simulink model "Simulink_Simulink_PIL_Cruise_Crontrol_r2020b"  (R2024a)
settings: Solver=VariableStepAuto  StartTime=0.0  StopTime=Tsim  FixedStep=Ts/20  RelTol=1e-3
values from neighbouring files (symbols this model uses):
  noise = 0    [main_Simulink_PIL_Cruise_Crontrol.m]
  PIL = 1    [main_Simulink_PIL_Cruise_Crontrol.m]
  Ts = 1/fs    (= 0.01)    [main_Simulink_PIL_Cruise_Crontrol.m]
undefined symbols (not defined in the file or in its folder): g
libraries: aerolibactuator x2, aerolibatmos2 x2, simulink x1
settings Model: SimulationMode=accelerator  Creator=ricardo  LastModifiedBy=mason
settings SolverCC: AlgebraicLoopSolver=TrustRegion
settings DataIOCC: ReturnWorkspaceOutputs=off
settings DebuggingCC: UnconnectedInputMsg=warning  UnconnectedOutputMsg=warning  UnconnectedLineMsg=warning  ArithmeticOperatorsInVariantConditions=warning
settings ModelReferenceCC: EnableRefExpFcnMdlSchedulingChecks=on
settings SFSimCC: CustomCodeUndefinedFunction=UseInterfaceOnly
settings RTWCC: GPUComputeCapability=3.5  DLArmComputeVersion=19.05

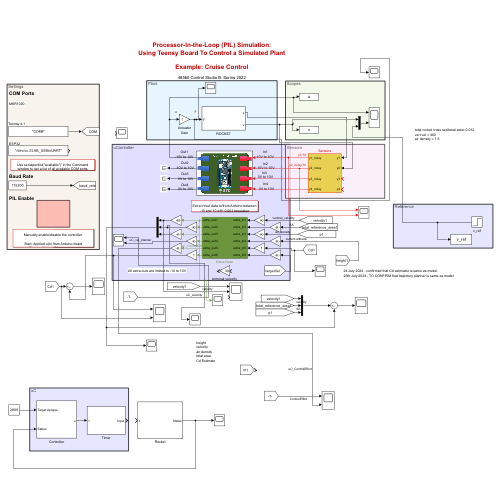
[thumbnail: Simulink's stored preview of the top-level diagram]
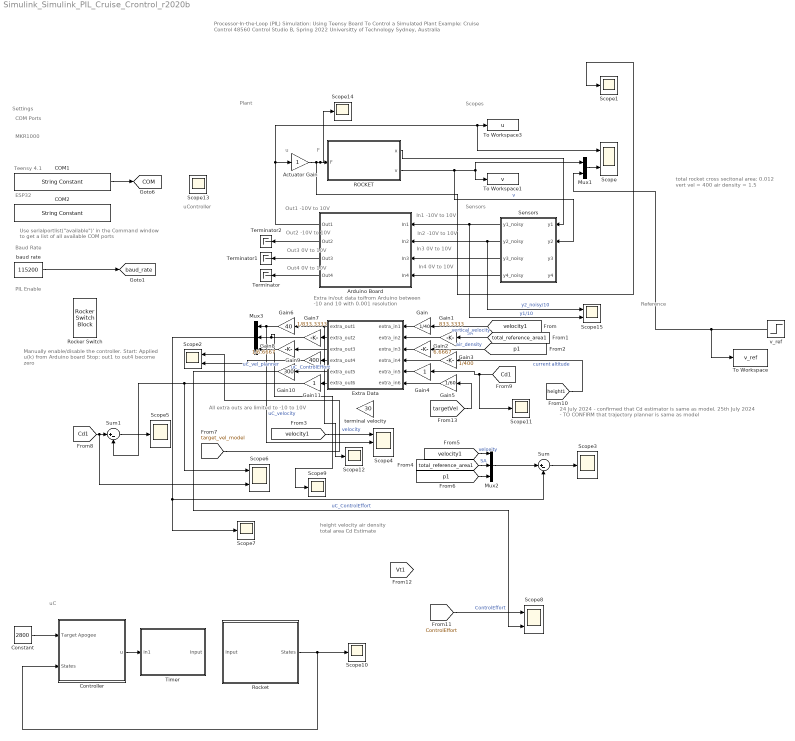
== system Simulink_Simulink_PIL_Cruise_Crontrol_r2020b ==
  note: 24 July 2024 - confirmed that Cd estimator is same as model.
      | 25th July 2024 - TO CONFIRM that trajectory planner is same as model
  note: All extra outs are limited to -10 to 10V
  note: height
      | velocity
      | air density
      | total area
      | Cd Estimate
  note: total rocket cross secitonal area: 0.012
      | vert vel = 400
      | air density = 1.5
  note: F
  note: u
  note: MKR1000
  note: COM Ports
  note: Settings
  note: Scopes
  note: Plant
  note: Reference
  note: Sensors
  note: uController
  note: Out1
      | -10V to 10V
  note: Processor-In-the-Loop (PIL) Simulation:
      | Using Teensy Board To Control a Simulated Plant
      |
      | Example: Cruise Control
      |
      | 48560 Control Studio B, Spring 2022
      | Universitty of Technology Sydney, Australia
  note: Out2
      | -10V to 10V
  note: Out3
      | 0V to 10V
  note: Out4
      | 0V to 10V
  note: In1
      | -10V to 10V
  note: In2
      | -10V to 10V
  note: In3
      | 0V to 10V
  note: In4
      | 0V to 10V
  note: Manually enable/disable the controller.
      |
      | Start: Applied u(k) from Arduino board
      | Stop: out1 to out4 become zero
  note: Extra in/out data to/from Arduino between -10 and 10 with 0.001 resolution
  note: Baud Rate
  note: PIL Enable
  note: Use serialportlist("available")' in the Command window to get a list of all available COM ports
  note: ESP32
  note: Teensy 4.1
  note: uC
  Actuator Gain : Gain
  Arduino Board : Subsystem
      mask Display: image('$imagefile'); % Use "Edit Image" on toolstrip to change.
  COM1 : StringConstant  String="\"COM8\""
  COM2 : StringConstant  String="\"/dev/cu.SLAB_USBtoUART\""
  Constant : Constant  Value=2800
  Controller : Subsystem
  Extra Data : Subsystem
  Gain : Gain  Gain=1/40
  Gain1 : Gain  Gain=833.3333
  Gain10 : Gain  Gain=300
  Gain11 : Gain
  Gain2 : Gain  Gain=6.6667
  Gain3 : Gain  Gain=1/400
  Gain4 : Gain
  Gain5 : Gain  Gain=1/60
  Gain6 : Gain  Gain=40
  Gain7 : Gain  Gain=1/833.3333
  Gain8 : Gain  Gain=1/6.6667
  Gain9 : Gain  Gain=400
  Mux1 : Mux  Inputs=2
  Mux2 : Mux  Inputs=3
  Mux3 : Mux  Inputs=3
  ROCKET : Subsystem
  Rocker Switch : RockerSwitchBlock  LabelPosition=Hide
      settings: Values={{'Stop', 'Start'}, [0 1]}
  Rocket : Subsystem
  Scope{,2,6,8,15} (5 alike) : Scope  NumInputPorts=2
  Scope{1,3,5,7,9..14} (10 alike) : Scope
  Scope4 : Scope  NumInputPorts=3
  Sensors : Subsystem
  Sum : Sum  Inputs=|+-
  Sum1 : Sum  Inputs=|+-
  Terminator : Terminator
  Terminator1 : Terminator
  Terminator2 : Terminator
  Timer : Subsystem
  To Workspace : ToWorkspace  VariableName=v_ref  SampleTime=Ts/20
  To Workspace1 : ToWorkspace  VariableName=v  SampleTime=Ts/20
  To Workspace3 : ToWorkspace  VariableName=u  SampleTime=Ts/20
  baud rate : Constant  Value=115200
  terminal velocity : Gain  Gain=30
  v_ref : Step  Time=0.001  After=2800  SampleTime=0
  tag scope: COM=global, baud_rate=global
  wires:
  Arduino Board/2(Out2) -> Terminator2/1
  Arduino Board/3(Out3) -> Terminator1/1
  Arduino Board/4(Out4) -> Terminator/1
  Extra Data/1(extra_out1) -> Gain6/1, Scope12/1
  Extra Data/3(extra_out3) -> Gain8/1
  Sensors/1(y1_noisy) -> Scope15/2, Arduino Board/1(In1)  "y1/10"
  Sensors/4(y4_noisy) -> Arduino Board/4(In4)
  baud rate/1 -> [baud_rate]
  Sensors/2(y2_noisy) -> Scope15/1, Arduino Board/2(In2)  "y2_noisy/10"
  Sensors/3(y3_noisy) -> Arduino Board/3(In3)
  v_ref/1 -> To Workspace/1, Mux1/2
  ROCKET/2(v) -> Mux1/1, To Workspace1/1, Sensors/2(y2)  "v"
  ROCKET/1(x) -> Sensors/1(y1)
  Actuator Gain/1 -> Scope14/1, ROCKET/1(F), Scope1/1
  Mux1/1 -> Scope/2
  COM1/1 -> [COM]
  Rocket/1(States) -> Scope10/1, Controller/2(States)
  Constant/1 -> Controller/1(Target Apogee)
  Controller/1(u) -> Timer/1(In1)
  Gain/1 -> Extra Data/1(extra_in1)
  Gain1/1 -> Extra Data/2(extra_in2)
  Gain2/1 -> Extra Data/3(extra_in3)
  Gain4/1 -> Extra Data/5(extra_in5)
  Gain3/1 -> Extra Data/4(extra_in4)
  Gain5/1 -> Extra Data/6(extra_in6)
  Gain9/1 -> Scope2/2  "uC_vel_planner"
  Gain8/1 -> Mux3/3
  Gain6/1 -> Scope4/2, Mux3/1  "uC_velocity"
  Extra Data/2(extra_out2) -> Gain7/1
  Extra Data/4(extra_out4) -> Gain9/1
  Extra Data/6(extra_out6) -> Gain11/1
  [total_reference_area1] -> Gain1/1  "SA"
  [velocity1] -> Gain/1  "vertical_velocity"
  [p1] -> Gain2/1  "air_density"
  [velocity1] -> Mux2/1  "velocity"
  [total_reference_area1] -> Mux2/2  "SA"
  [p1] -> Mux2/3
  Mux2/1 -> Sum/1
  Mux3/1 -> Scope7/1, Sum/2
  Sum/1 -> Scope3/1
  [velocity1] -> Scope4/1  "velocity"
  [Cd1] -> Scope6/2, Sum1/1
  Gain11/1 -> Scope6/1, Sum1/2
  Sum1/1 -> Scope5/1
  [height1] -> Gain3/1  "current altitude"
  [target_vel_model] -> Scope2/1
  Extra Data/5(extra_out5) -> Gain10/1  "uC_ControlEffort"
  Gain7/1 -> Scope9/1, Mux3/2
  [Cd1] -> Scope11/1, Gain4/1
  Arduino Board/1(Out1) -> Scope/1, To Workspace3/1, Actuator Gain/1
  [ControlEffort] -> Scope8/1  "ControlEffort"
  Gain10/1 -> Scope8/2  "uC_ControlEffort"
  [targetVel] -> Gain5/1

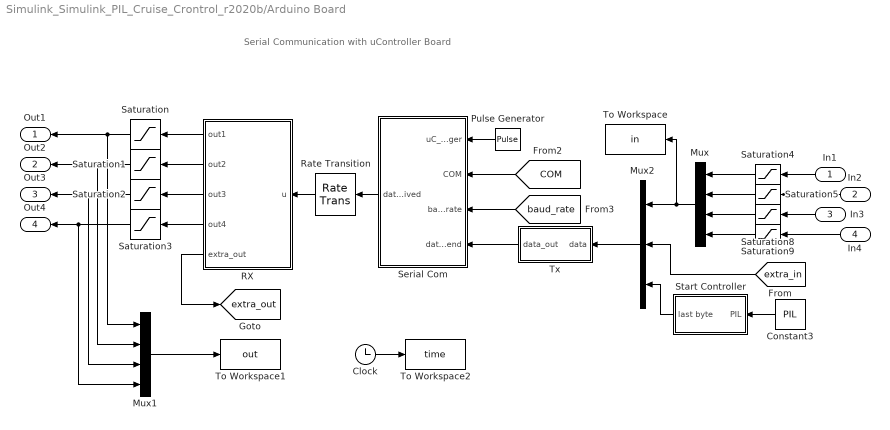
== system Simulink_Simulink_PIL_Cruise_Crontrol_r2020b/Arduino Board ==
  note: Serial Communication with uController Board
  In1 : Inport
  In2 : Inport  Port=2
  In3 : Inport  Port=3
  In4 : Inport  Port=4
  Clock : Clock
  Constant3 : Constant  Value=PIL
  Mux : Mux
  Mux1 : Mux
  Mux2 : Mux  Inputs=3
  Pulse Generator : DiscretePulseGenerator  PulseType=Time based  Period=Ts  PulseWidth=50
  RX : MATLAB Function  TreatAsAtomicUnit=on
  Rate Transition : RateTransition  InitialCondition=zeros(21,1)
  Saturation{,1,4..5} (4 alike) : Saturate  UpperLimit=10  LowerLimit=-10
  Saturation{2..3,8..9} (4 alike) : Saturate  UpperLimit=10  LowerLimit=0
  Serial Com : MATLAB Function  TreatAsAtomicUnit=on  SystemSampleTime=Ts/10
  Start Controller : Subsystem
  To Workspace : ToWorkspace  VariableName=in  SampleTime=Ts/20
  To Workspace1 : ToWorkspace  VariableName=out  SampleTime=Ts/20
  To Workspace2 : ToWorkspace  VariableName=time  SampleTime=Ts/20
  Tx : MATLAB Function  TreatAsAtomicUnit=on  SystemSampleTime=Ts/10
  Out1 : Outport  VectorParamsAs1DForOutWhenUnconnected=off
  Out2 : Outport  Port=2  VectorParamsAs1DForOutWhenUnconnected=off
  Out3 : Outport  Port=3  VectorParamsAs1DForOutWhenUnconnected=off
  Out4 : Outport  Port=4  VectorParamsAs1DForOutWhenUnconnected=off
  tag scope: extra_out=global
  wires:
  RX/1(out1) -> Saturation/1
  RX/2(out2) -> Saturation1/1
  RX/3(out3) -> Saturation2/1
  Mux1/1 -> To Workspace1/1
  Clock/1 -> To Workspace2/1
  Saturation/1 -> Out1/1, Mux1/1
  Saturation1/1 -> Out2/1, Mux1/2
  Saturation2/1 -> Out3/1, Mux1/3
  Saturation3/1 -> Out4/1, Mux1/4
  RX/4(out4) -> Saturation3/1
  RX/5(extra_out) -> [extra_out]
  Mux/1 -> Mux2/1, To Workspace/1
  [COM] -> Serial Com/2(COM)
  [baud_rate] -> Serial Com/3(baud_rate)
  Pulse Generator/1 -> Serial Com/1(uC_trigger)
  Serial Com/1(data_received) -> Rate Transition/1
  Rate Transition/1 -> RX/1(u)
  Constant3/1 -> Start Controller/1(PIL)
  In1/1 -> Saturation4/1
  In2/1 -> Saturation5/1
  In3/1 -> Saturation8/1
  In4/1 -> Saturation9/1
  Saturation4/1 -> Mux/1
  Saturation5/1 -> Mux/2
  Saturation8/1 -> Mux/3
  Saturation9/1 -> Mux/4
  [extra_in] -> Mux2/2
  Start Controller/1(last byte) -> Mux2/3
  Mux2/1 -> Tx/1(data)
  Tx/1(data_out) -> Serial Com/4(data_send)

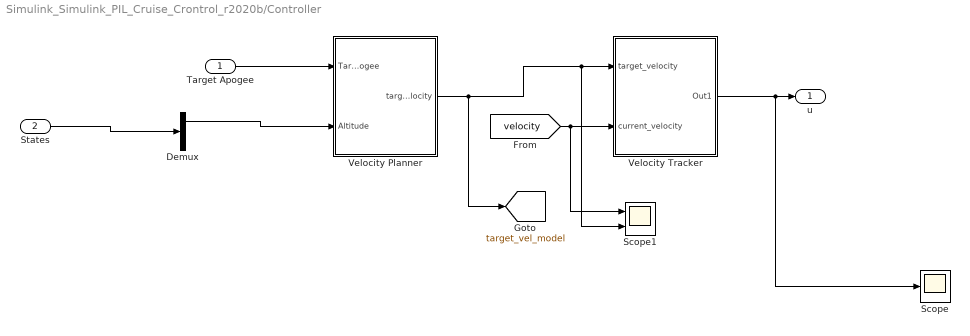
== system Simulink_Simulink_PIL_Cruise_Crontrol_r2020b/Controller ==
  Target Apogee : Inport
  States : Inport  Port=2
  Demux : Demux  Outputs=5
  Scope : Scope
  Scope1 : Scope  NumInputPorts=2
  Velocity Planner : Subsystem
  Velocity Tracker : Subsystem
  u : Outport
  tag scope: target_vel_model=global
  wires:
  Target Apogee/1 -> Velocity Planner/1(Target Apogee)
  Velocity Tracker/1(Out1) -> Scope/1, u/1
  [velocity] -> Scope1/1, Velocity Tracker/2(current_velocity)
  Velocity Planner/1(target_velocity) -> [target_vel_model], Scope1/2, Velocity Tracker/1(target_velocity)
  States/1 -> Demux/1
  Demux/1 -> Velocity Planner/2(Altitude)

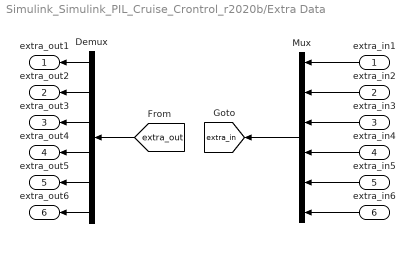
== system Simulink_Simulink_PIL_Cruise_Crontrol_r2020b/Extra Data ==
  extra_in1 : Inport
  extra_in2 : Inport  Port=2
  extra_in3 : Inport  Port=3
  extra_in4 : Inport  Port=4
  extra_in5 : Inport  Port=5
  extra_in6 : Inport  Port=6
  Demux : Demux  Outputs=6
  Mux : Mux  Inputs=6
  extra_out1 : Outport
  extra_out2 : Outport  Port=2
  extra_out3 : Outport  Port=3
  extra_out4 : Outport  Port=4
  extra_out5 : Outport  Port=5
  extra_out6 : Outport  Port=6
  tag scope: extra_in=global
  wires:
  extra_in4/1 -> Mux/4
  extra_in3/1 -> Mux/3
  extra_in2/1 -> Mux/2
  extra_in1/1 -> Mux/1
  Mux/1 -> [extra_in]
  [extra_out] -> Demux/1
  Demux/1 -> extra_out1/1
  Demux/2 -> extra_out2/1
  Demux/3 -> extra_out3/1
  Demux/4 -> extra_out4/1
  extra_in5/1 -> Mux/5
  extra_in6/1 -> Mux/6
  Demux/6 -> extra_out6/1
  Demux/5 -> extra_out5/1

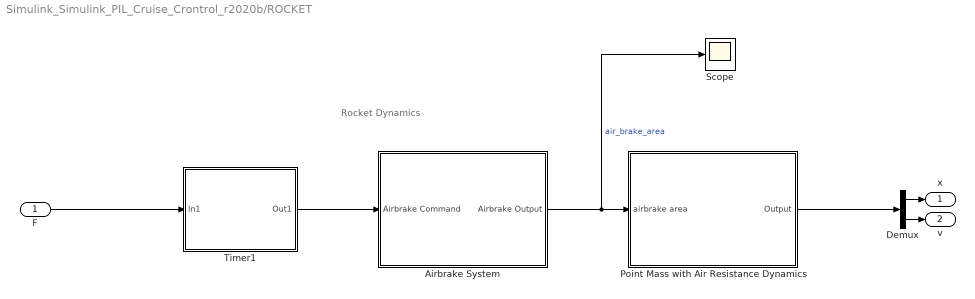
== system Simulink_Simulink_PIL_Cruise_Crontrol_r2020b/ROCKET ==
  note: Rocket Dynamics
  F : Inport
  Airbrake System : Subsystem
      mask Display: image('airbrake.png');
  Demux : Demux  Outputs=2
  "Point Mass with Air Resistance Dynamics " : Subsystem
      mask Display: image('rocket.jpeg');
  Scope : Scope
  Timer1 : Subsystem
  x : Outport  VectorParamsAs1DForOutWhenUnconnected=off
  v : Outport  Port=2  VectorParamsAs1DForOutWhenUnconnected=off
  wires:
  Airbrake System/1(Airbrake Output) -> Scope/1, "Point Mass with Air Resistance Dynamics "/1(airbrake area)  "air_brake_area"
  F/1 -> Timer1/1(In1)
  "Point Mass with Air Resistance Dynamics "/1(Output) -> Demux/1
  Demux/1 -> x/1
  Demux/2 -> v/1
  Timer1/1(Out1) -> Airbrake System/1(Airbrake Command)

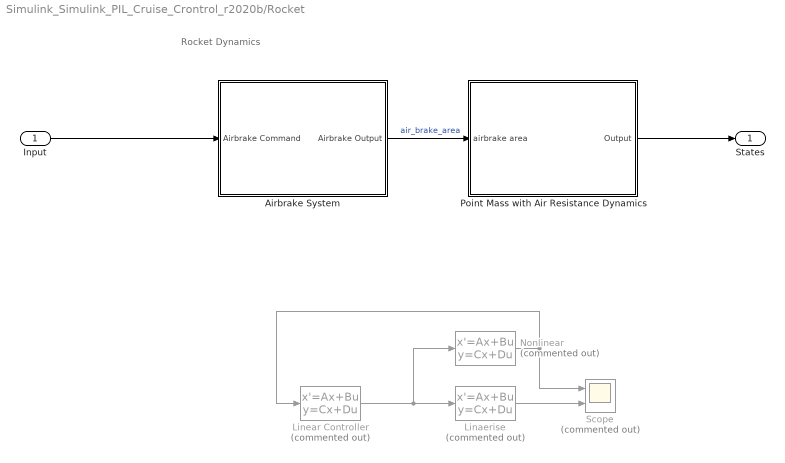
== system Simulink_Simulink_PIL_Cruise_Crontrol_r2020b/Rocket ==
  note: Rocket Dynamics
  Input : Inport
  Airbrake System : Subsystem
      mask Display: image('airbrake.png');
  "Linaerise " : StateSpace  Commented=on  InitialCondition=0
  Linear Controller : StateSpace  Commented=on  InitialCondition=0
  Nonlinear : StateSpace  Commented=on  InitialCondition=0
  "Point Mass with Air Resistance Dynamics " : Subsystem
      mask Display: image('rocket.jpeg');
  Scope : Scope  Commented=on  NumInputPorts=2
  States : Outport
  wires:
  "Point Mass with Air Resistance Dynamics "/1(Output) -> States/1
  Linear Controller/1 -> Nonlinear/1, "Linaerise "/1
  Nonlinear/1 -> Linear Controller/1, Scope/1
  "Linaerise "/1 -> Scope/2
  Input/1 -> Airbrake System/1(Airbrake Command)
  Airbrake System/1(Airbrake Output) -> "Point Mass with Air Resistance Dynamics "/1(airbrake area)  "air_brake_area"

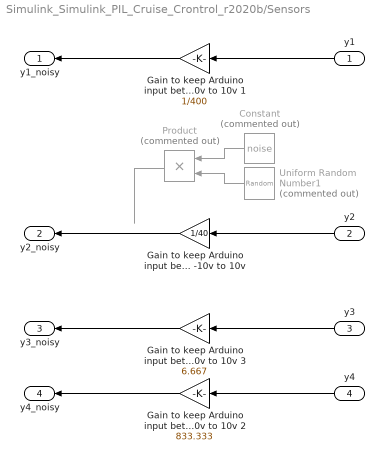
== system Simulink_Simulink_PIL_Cruise_Crontrol_r2020b/Sensors ==
  y1 : Inport
  y2 : Inport  Port=2
  y3 : Inport  Port=3
  y4 : Inport  Port=4
  Constant : Constant  Commented=on  Value=noise
  "Gain to keep Arduino input between -10v to 10v " : Gain  Gain=1/40
  Gain to keep Arduino input between -10v to 10v 1 : Gain  Gain=1/400
  Gain to keep Arduino input between -10v to 10v 2 : Gain  Gain=833.333
  Gain to keep Arduino input between -10v to 10v 3 : Gain  Gain=6.667
  Product : Product  Commented=on
  Uniform Random Number1 : UniformRandomNumber  Commented=on  Minimum=-0.1  Maximum=0.1  SampleTime=0.5*Ts
  y1_noisy : Outport  VectorParamsAs1DForOutWhenUnconnected=off
  y2_noisy : Outport  Port=2  VectorParamsAs1DForOutWhenUnconnected=off
  y3_noisy : Outport  Port=3  VectorParamsAs1DForOutWhenUnconnected=off
  y4_noisy : Outport  Port=4  VectorParamsAs1DForOutWhenUnconnected=off
  wires:
  y2/1 -> "Gain to keep Arduino input between -10v to 10v "/1
  y3/1 -> Gain to keep Arduino input between -10v to 10v 3/1
  y4/1 -> Gain to keep Arduino input between -10v to 10v 2/1
  y1/1 -> Gain to keep Arduino input between -10v to 10v 1/1
  Uniform Random Number1/1 -> Product/2
  Product/1 -> ?
  Constant/1 -> Product/1
  "Gain to keep Arduino input between -10v to 10v "/1 -> y2_noisy/1
  Gain to keep Arduino input between -10v to 10v 1/1 -> y1_noisy/1
  Gain to keep Arduino input between -10v to 10v 2/1 -> y4_noisy/1
  Gain to keep Arduino input between -10v to 10v 3/1 -> y3_noisy/1

== system Simulink_Simulink_PIL_Cruise_Crontrol_r2020b/Timer ==
  In1 : Inport
  Clock : Clock
  Constant1 : Constant  Value=0
  Switch : Switch  Criteria=u2 > Threshold  Threshold=5  SaturateOnIntegerOverflow=off  InputSameDT=off
  Input : Outport
  wires:
  Switch/1 -> Input/1
  Clock/1 -> Switch/2
  In1/1 -> Switch/1
  Constant1/1 -> Switch/3

== system Simulink_Simulink_PIL_Cruise_Crontrol_r2020b/Arduino Board/Start Controller ==
  PIL : Inport
  Constant : Constant  Value=0
  Constant1 : Constant  Value=255
  Switch : Switch  Criteria=u2 > Threshold  SaturateOnIntegerOverflow=off  InputSameDT=off
  last byte : Outport
  wires:
  Switch/1 -> last byte/1
  PIL/1 -> Switch/2
  Constant1/1 -> Switch/1
  Constant/1 -> Switch/3

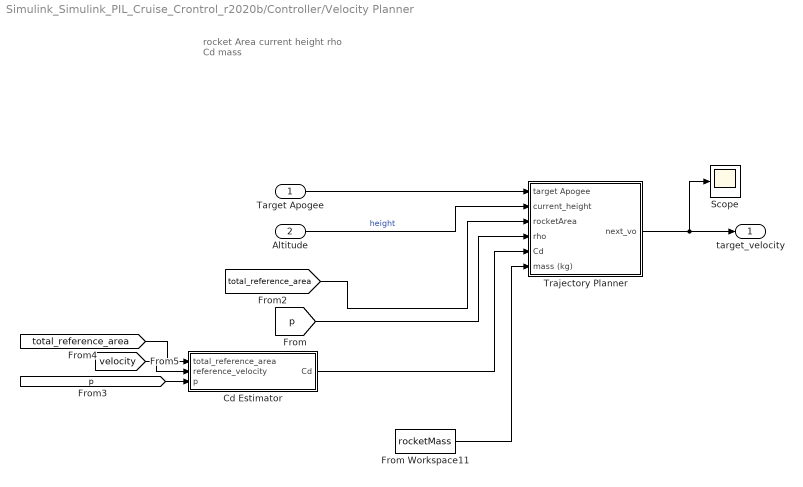
== system Simulink_Simulink_PIL_Cruise_Crontrol_r2020b/Controller/Velocity Planner ==
  note: rocket Area
      | current height
      | rho
      | Cd
      | mass
  Target Apogee : Inport
  Altitude : Inport  Port=2
  Cd Estimator : Subsystem
  From Workspace11 : FromWorkspace  VariableName=rocketMass
  Scope : Scope
  Trajectory Planner : Subsystem
  target_velocity : Outport
  wires:
  Altitude/1 -> Trajectory Planner/2(current_height)  "height"
  Target Apogee/1 -> Trajectory Planner/1(target Apogee)
  [p] -> Trajectory Planner/4(rho)
  From Workspace11/1 -> Trajectory Planner/6(mass (kg))
  [p] -> Cd Estimator/3(p)
  [velocity] -> Cd Estimator/2(reference_velocity)
  [total_reference_area] -> Cd Estimator/1(total_reference_area)
  [total_reference_area] -> Trajectory Planner/3(rocketArea)
  Trajectory Planner/1(next_vo) -> Scope/1, target_velocity/1
  Cd Estimator/1(Cd) -> Trajectory Planner/5(Cd)

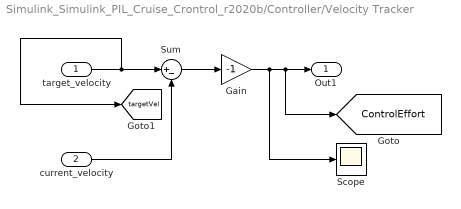
== system Simulink_Simulink_PIL_Cruise_Crontrol_r2020b/Controller/Velocity Tracker ==
  target_velocity : Inport
  current_velocity : Inport  Port=2
  Gain : Gain  Gain=-1
  Scope : Scope
  Sum : Sum  Inputs=|+-
  Out1 : Outport
  tag scope: ControlEffort=global, targetVel=global
  wires:
  Gain/1 -> Scope/1, [ControlEffort], Out1/1
  target_velocity/1 -> [targetVel], Sum/1
  current_velocity/1 -> Sum/2
  Sum/1 -> Gain/1

== system Simulink_Simulink_PIL_Cruise_Crontrol_r2020b/ROCKET/Airbrake System ==
  Airbrake Command : Inport
  Nonlinear Second-Order Actuator : aerolibactuator/Nonlinear Second-Order Actuator  wn_fin=10  z_fin=0.7  fin_max=maxAirbrakeArea  fin_min=0  fin_maxrate=0.4  fin_act_0=0  fin_act_vel=0
  Scope : Scope  NumInputPorts=2
  Scope1 : Scope
  Square Wave Generator : SignalGenerator  Commented=on  WaveForm=square  Amplitude=0.01  Units=rad/sec
  Airbrake Output : Outport
  wires:
  Nonlinear Second-Order Actuator/1 -> Scope1/1, Scope/2, Airbrake Output/1
  Airbrake Command/1 -> Nonlinear Second-Order Actuator/1, Scope/1

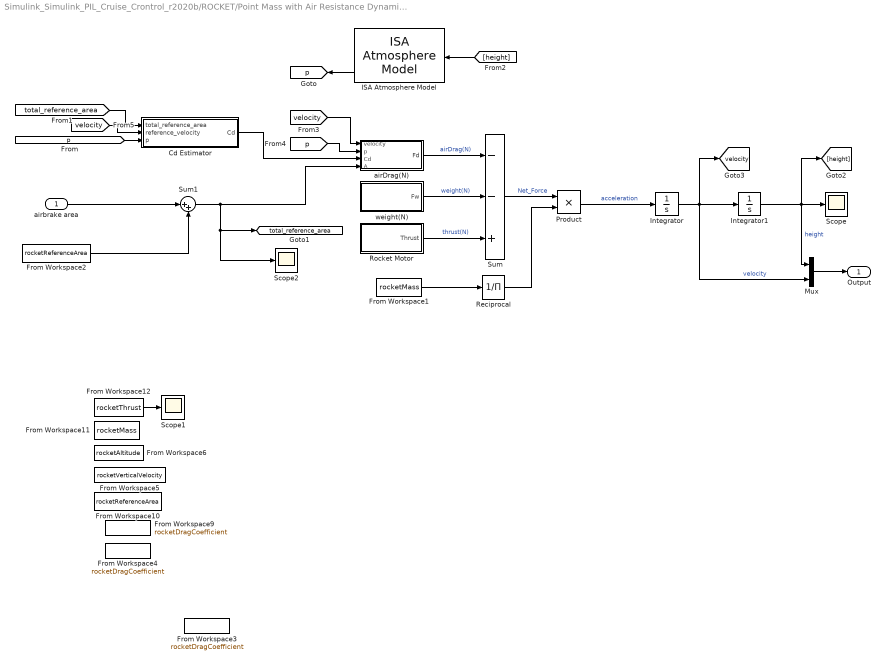
== system Simulink_Simulink_PIL_Cruise_Crontrol_r2020b/ROCKET/Point Mass with Air Resistance Dynamics  ==
  airbrake area : Inport
  Cd Estimator : Subsystem
  From Workspace1 : FromWorkspace  VariableName=rocketMass
  From Workspace10 : FromWorkspace  VariableName=rocketReferenceArea
  From Workspace11 : FromWorkspace  VariableName=rocketMass
  From Workspace12 : FromWorkspace  VariableName=rocketThrust
  From Workspace2 : FromWorkspace  VariableName=rocketReferenceArea
  From Workspace3 : FromWorkspace  VariableName=rocketDragCoefficient
  From Workspace4 : FromWorkspace  VariableName=rocketDragCoefficient
  From Workspace5 : FromWorkspace  VariableName=rocketVerticalVelocity
  From Workspace6 : FromWorkspace  VariableName=rocketAltitude
  From Workspace9 : FromWorkspace  VariableName=rocketDragCoefficient
  ISA Atmosphere Model : aerolibatmos2/ISA Atmosphere Model  useExtended=off  action=Warning  custom=off  viscosityOut=off  g=9.80665  gamma=1.4  R=287.0531  L=0.0065  h_trop=11000  h_strat=20000  rho0=1.225  P0=101325  T0=288.15  h0=0  S=110.4  Tref=273.15  muref=1.716e-5
  Integrator : Integrator
  Integrator1 : Integrator
  Mux : Mux  Inputs=2
  Product : Product
  Reciprocal : Product  Inputs=/
  "Rocket Motor " : Subsystem
  Scope : Scope
  Scope1 : Scope
  Scope2 : Scope
  Sum : Sum  Inputs=--+
  Sum1 : Sum  Inputs=|++
  airDrag(N) : Subsystem
  weight(N) : Subsystem
  Output : Outport
  tag scope: p=global, total_reference_area=global, velocity=global
  wires:
  "Rocket Motor "/1(Thrust) -> Sum/3  "thrust(N)"
  airDrag(N)/1(Fd) -> Sum/1  "airDrag(N)"
  weight(N)/1(Fw) -> Sum/2  "weight(N)"
  Sum/1 -> Product/1  "Net_Force"
  [p] -> Cd Estimator/3(p)
  ISA Atmosphere Model/4 -> [p]
  [total_reference_area] -> Cd Estimator/1(total_reference_area)
  [height] -> ISA Atmosphere Model/1
  [velocity] -> airDrag(N)/1(velocity)
  [p] -> airDrag(N)/2(p)
  Product/1 -> Integrator/1  "acceleration"
  Integrator/1 -> [velocity], Integrator1/1, Mux/2  "velocity"
  Integrator1/1 -> Mux/1, [height], Scope/1  "height"
  Mux/1 -> Output/1
  [velocity] -> Cd Estimator/2(reference_velocity)
  Reciprocal/1 -> Product/2
  From Workspace1/1 -> Reciprocal/1
  From Workspace12/1 -> Scope1/1
  airbrake area/1 -> Sum1/1
  Sum1/1 -> Scope2/1, [total_reference_area], airDrag(N)/4(A)
  From Workspace2/1 -> Sum1/2
  Cd Estimator/1(Cd) -> airDrag(N)/3(Cd)

== system Simulink_Simulink_PIL_Cruise_Crontrol_r2020b/ROCKET/Timer1 ==
  In1 : Inport
  Clock : Clock
  Constant1 : Constant  Value=0
  Switch : Switch  Criteria=u2 > Threshold  Threshold=5  SaturateOnIntegerOverflow=off  InputSameDT=off
  Out1 : Outport
  wires:
  Switch/1 -> Out1/1
  Clock/1 -> Switch/2
  In1/1 -> Switch/1
  Constant1/1 -> Switch/3

== system Simulink_Simulink_PIL_Cruise_Crontrol_r2020b/Rocket/Airbrake System ==
  Airbrake Command : Inport
  Nonlinear Second-Order Actuator : aerolibactuator/Nonlinear Second-Order Actuator  wn_fin=10  z_fin=0.7  fin_max=maxAirbrakeArea  fin_min=0  fin_maxrate=0.4  fin_act_0=0  fin_act_vel=0
  Scope : Scope  NumInputPorts=2
  Scope1 : Scope
  Square Wave Generator : SignalGenerator  Commented=on  WaveForm=square  Amplitude=0.01  Units=rad/sec
  Airbrake Output : Outport
  wires:
  Nonlinear Second-Order Actuator/1 -> Scope1/1, Scope/2, Airbrake Output/1
  Airbrake Command/1 -> Nonlinear Second-Order Actuator/1, Scope/1

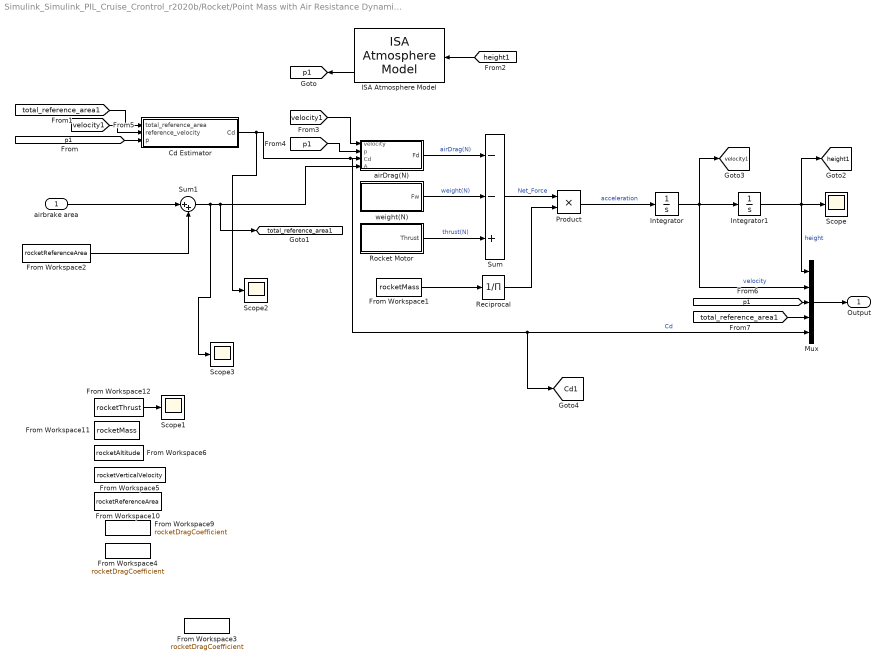
== system Simulink_Simulink_PIL_Cruise_Crontrol_r2020b/Rocket/Point Mass with Air Resistance Dynamics  ==
  airbrake area : Inport
  Cd Estimator : Subsystem
  From Workspace1 : FromWorkspace  VariableName=rocketMass
  From Workspace10 : FromWorkspace  VariableName=rocketReferenceArea
  From Workspace11 : FromWorkspace  VariableName=rocketMass
  From Workspace12 : FromWorkspace  VariableName=rocketThrust
  From Workspace2 : FromWorkspace  VariableName=rocketReferenceArea
  From Workspace3 : FromWorkspace  VariableName=rocketDragCoefficient
  From Workspace4 : FromWorkspace  VariableName=rocketDragCoefficient
  From Workspace5 : FromWorkspace  VariableName=rocketVerticalVelocity
  From Workspace6 : FromWorkspace  VariableName=rocketAltitude
  From Workspace9 : FromWorkspace  VariableName=rocketDragCoefficient
  ISA Atmosphere Model : aerolibatmos2/ISA Atmosphere Model  useExtended=off  action=Warning  custom=off  viscosityOut=off  g=9.80665  gamma=1.4  R=287.0531  L=0.0065  h_trop=11000  h_strat=20000  rho0=1.225  P0=101325  T0=288.15  h0=0  S=110.4  Tref=273.15  muref=1.716e-5
  Integrator : Integrator
  Integrator1 : Integrator
  Mux : Mux  Inputs=5
  Product : Product
  Reciprocal : Product  Inputs=/
  "Rocket Motor " : Subsystem
  Scope{,1..3} (4 alike) : Scope
  Sum : Sum  Inputs=--+
  Sum1 : Sum  Inputs=|++
  airDrag(N) : Subsystem
  weight(N) : Subsystem
  Output : Outport
  tag scope: Cd1=global, height1=global, p1=global, total_reference_area1=global, velocity1=global
  wires:
  "Rocket Motor "/1(Thrust) -> Sum/3  "thrust(N)"
  airDrag(N)/1(Fd) -> Sum/1  "airDrag(N)"
  weight(N)/1(Fw) -> Sum/2  "weight(N)"
  Sum/1 -> Product/1  "Net_Force"
  [p1] -> Cd Estimator/3(p)
  ISA Atmosphere Model/4 -> [p1]
  [total_reference_area1] -> Cd Estimator/1(total_reference_area)
  [height1] -> ISA Atmosphere Model/1
  [velocity1] -> airDrag(N)/1(velocity)
  [p1] -> airDrag(N)/2(p)
  Product/1 -> Integrator/1  "acceleration"
  Integrator/1 -> [velocity1], Integrator1/1, Mux/2  "velocity"
  Integrator1/1 -> Mux/1, [height1], Scope/1  "height"
  Mux/1 -> Output/1
  [velocity1] -> Cd Estimator/2(reference_velocity)
  Reciprocal/1 -> Product/2
  From Workspace1/1 -> Reciprocal/1
  From Workspace12/1 -> Scope1/1
  airbrake area/1 -> Sum1/1
  Sum1/1 -> Scope3/1, [total_reference_area1], airDrag(N)/4(A)
  From Workspace2/1 -> Sum1/2
  Cd Estimator/1(Cd) -> Scope2/1, [Cd1], Mux/5, airDrag(N)/3(Cd)  "Cd"
  [p1] -> Mux/3
  [total_reference_area1] -> Mux/4

== system Simulink_Simulink_PIL_Cruise_Crontrol_r2020b/Controller/Velocity Planner/Cd Estimator ==
  total_reference_area : Inport
  reference_velocity : Inport  Port=2
  p : Inport  Port=3
  Rocket Specific Cd Estimator : MATLAB Function  TreatAsAtomicUnit=on
  Cd : Outport
  wires:
  Rocket Specific Cd Estimator/1(Cd) -> Cd/1
  total_reference_area/1 -> Rocket Specific Cd Estimator/1(SA)
  reference_velocity/1 -> Rocket Specific Cd Estimator/2(V)
  p/1 -> Rocket Specific Cd Estimator/3(rho)

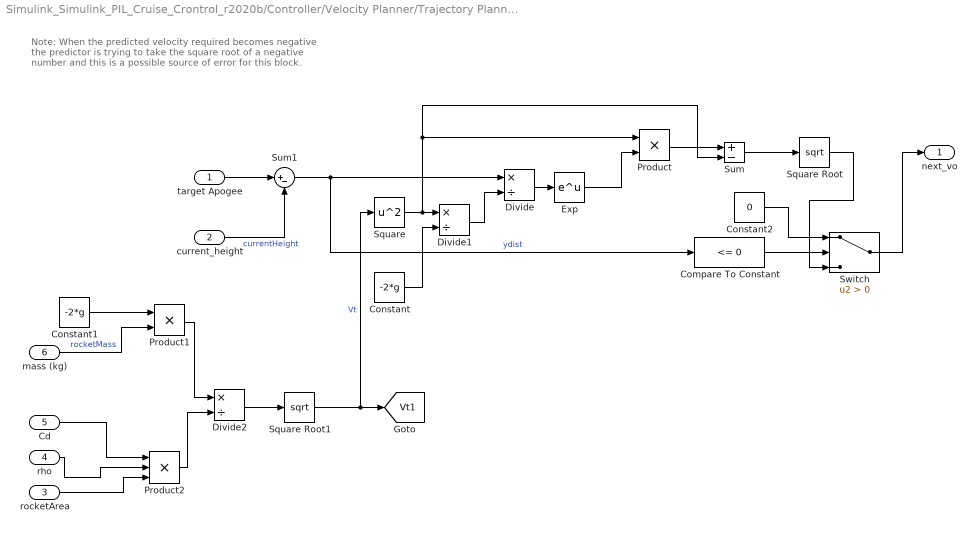
== system Simulink_Simulink_PIL_Cruise_Crontrol_r2020b/Controller/Velocity Planner/Trajectory Planner ==
  note: Note: When the predicted velocity required becomes negative the predictor is trying to take the square root of a negative number and this is a possible source of error for this block.
  target Apogee : Inport
  current_height : Inport  Port=2
  rocketArea : Inport  Port=3
  rho : Inport  Port=4
  Cd : Inport  Port=5
  mass (kg) : Inport  Port=6
  Compare To Constant : simulink/Logic and Bit Operations/Compare To Constant  relop=<=  const=0  OutDataTypeStr=boolean
  Constant : Constant  Value=-2*g
  Constant1 : Constant  Value=-2*g
  Constant2 : Constant  Value=0
  Divide : Product  Inputs=*/
  Divide1 : Product  Inputs=*/
  Divide2 : Product  Inputs=*/
  Exp : Math
  Product : Product
  Product1 : Product
  Product2 : Product  Inputs=3
  Square : Math  Operator=square
  Square Root : Sqrt
  Square Root1 : Sqrt
  Sum : Sum  Inputs=+-
  Sum1 : Sum  Inputs=|+-
  Switch : Switch  Criteria=u2 > Threshold  SaturateOnIntegerOverflow=off  InputSameDT=off
  next_vo : Outport
  tag scope: Vt1=global
  wires:
  Sum/1 -> Square Root/1
  Product/1 -> Sum/1
  Exp/1 -> Product/2
  Divide/1 -> Exp/1
  Sum1/1 -> Compare To Constant/1, Divide/1  "ydist"
  Constant/1 -> Divide1/2
  Divide1/1 -> Divide/2
  Square/1 -> Sum/2, Product/1, Divide1/1
  target Apogee/1 -> Sum1/1
  Product2/1 -> Divide2/2
  Square Root1/1 -> [Vt1], Square/1  "Vt"
  Cd/1 -> Product2/1
  Divide2/1 -> Square Root1/1
  rocketArea/1 -> Product2/3
  Product1/1 -> Divide2/1
  Constant1/1 -> Product1/1
  rho/1 -> Product2/2
  mass (kg)/1 -> Product1/2  "rocketMass"
  current_height/1 -> Sum1/2  "currentHeight"
  Compare To Constant/1 -> Switch/2
  Constant2/1 -> Switch/1
  Square Root/1 -> Switch/3
  Switch/1 -> next_vo/1

== system Simulink_Simulink_PIL_Cruise_Crontrol_r2020b/ROCKET/Point Mass with Air Resistance Dynamics /Cd Estimator ==
  total_reference_area : Inport
  reference_velocity : Inport  Port=2
  p : Inport  Port=3
  Rocket Specific Cd Estimator : MATLAB Function  TreatAsAtomicUnit=on
  Cd : Outport
  wires:
  Rocket Specific Cd Estimator/1(Cd) -> Cd/1
  total_reference_area/1 -> Rocket Specific Cd Estimator/1(SA)
  reference_velocity/1 -> Rocket Specific Cd Estimator/2(V)
  p/1 -> Rocket Specific Cd Estimator/3(rho)

== system Simulink_Simulink_PIL_Cruise_Crontrol_r2020b/ROCKET/Point Mass with Air Resistance Dynamics /Rocket Motor  ==
  From Workspace12 : FromWorkspace  VariableName=rocketThrust
  Thrust : Outport
  wires:
  From Workspace12/1 -> Thrust/1

== system Simulink_Simulink_PIL_Cruise_Crontrol_r2020b/ROCKET/Point Mass with Air Resistance Dynamics /airDrag(N) ==
  velocity : Inport
  p : Inport  Port=2
  Cd : Inport  Port=3
  A : Inport  Port=4
  Constant : Constant  Value=0.5
  Product : Product  Inputs=5
  Square : Math  Operator=square
  Fd : Outport
  wires:
  velocity/1 -> Square/1
  Square/1 -> Product/1  "v^2"
  p/1 -> Product/2  "p"
  Cd/1 -> Product/3  "Cd"
  A/1 -> Product/4  "A"
  Constant/1 -> Product/5
  Product/1 -> Fd/1  "Fd"

== system Simulink_Simulink_PIL_Cruise_Crontrol_r2020b/ROCKET/Point Mass with Air Resistance Dynamics /weight(N) ==
  From Workspace11 : FromWorkspace  VariableName=rocketMass
  gravity : Gain  Gain=9.80665
  Fw : Outport
  wires:
  From Workspace11/1 -> gravity/1
  gravity/1 -> Fw/1

== system Simulink_Simulink_PIL_Cruise_Crontrol_r2020b/Rocket/Point Mass with Air Resistance Dynamics /Cd Estimator ==
  total_reference_area : Inport
  reference_velocity : Inport  Port=2
  p : Inport  Port=3
  Rocket Specific Cd Estimator : MATLAB Function  TreatAsAtomicUnit=on
  Cd : Outport
  wires:
  Rocket Specific Cd Estimator/1(Cd) -> Cd/1
  total_reference_area/1 -> Rocket Specific Cd Estimator/1(SA)
  reference_velocity/1 -> Rocket Specific Cd Estimator/2(V)
  p/1 -> Rocket Specific Cd Estimator/3(rho)

== system Simulink_Simulink_PIL_Cruise_Crontrol_r2020b/Rocket/Point Mass with Air Resistance Dynamics /Rocket Motor  ==
  From Workspace12 : FromWorkspace  VariableName=rocketThrust
  Thrust : Outport
  wires:
  From Workspace12/1 -> Thrust/1

== system Simulink_Simulink_PIL_Cruise_Crontrol_r2020b/Rocket/Point Mass with Air Resistance Dynamics /airDrag(N) ==
  velocity : Inport
  p : Inport  Port=2
  Cd : Inport  Port=3
  A : Inport  Port=4
  Constant : Constant  Value=0.5
  Product : Product  Inputs=5
  Square : Math  Operator=square
  Fd : Outport
  wires:
  velocity/1 -> Square/1
  Square/1 -> Product/1  "v^2"
  p/1 -> Product/2  "p"
  Cd/1 -> Product/3  "Cd"
  A/1 -> Product/4  "A"
  Constant/1 -> Product/5
  Product/1 -> Fd/1  "Fd"

== system Simulink_Simulink_PIL_Cruise_Crontrol_r2020b/Rocket/Point Mass with Air Resistance Dynamics /weight(N) ==
  From Workspace11 : FromWorkspace  VariableName=rocketMass
  gravity : Gain  Gain=9.80665
  Fw : Outport
  wires:
  From Workspace11/1 -> gravity/1
  gravity/1 -> Fw/1

== matlab function Simulink_Simulink_PIL_Cruise_Crontrol_r2020b/Arduino Board/RX ==
  data: u input; out1 output; out2 output; out3 output; out4 output; extra_out output
%% Rx Data from uController Board
% 
%
% Control Studio A/B,
% The University of Technology Sydney (UTS)
% Sydney, NSW, Australia
%
% Dr Ricardo P. Aguilera
% August 2021
%%%%%%%%%%%%%%%%%%%%%%%%%%%%%%%%%%%%%%%%%%%%%%%%%%%%%%%%%%%%%%%%%%%%%%%%%%%%

function [out1, out2, out3, out4, extra_out] = fcn(u)
    [out1, out2, out3, out4, extra_out] = uC_Rx(u);
end

== matlab function Simulink_Simulink_PIL_Cruise_Crontrol_r2020b/Controller/Velocity Planner/Cd Estimator/Rocket Specific Cd Estimator ==
  data: SA input; Cd output; V input; rho input
function Cd = fcn(SA,V,rho)
u1 =  43.32270126;  % Total rocket SA.
u2 = -0.000687709; % Velocity
u3 = 0.531869262; % Air density
intercept = -0.447146101;
Cd = (SA*u1)+ (V*u2)+ (rho*u3) + (intercept) ;
end

== matlab function Simulink_Simulink_PIL_Cruise_Crontrol_r2020b/Arduino Board/Serial Com ==
  data: uC_trigger input; COM input; baud_rate input; data_received output; data_send input
%% Serial Communicaiton to/from uController Board
% 
%
% Control Studio A/B,
% The University of Technology Sydney (UTS)
% Sydney, NSW, Australia
%
% Dr Ricardo P. Aguilera
% August 2021
%%%%%%%%%%%%%%%%%%%%%%%%%%%%%%%%%%%%%%%%%%%%%%%%%%%%%%%%%%%%%%%%%%%%%%%%%%%%

function data_received  = fcn(uC_trigger, COM, baud_rate, data_send)
    data_received = uC_SerialCom(uC_trigger, COM, baud_rate, data_send);
end

== matlab function Simulink_Simulink_PIL_Cruise_Crontrol_r2020b/Arduino Board/Tx ==
  data: data input; data_out output
%% Data preconditioning to be sent to uController Board
% 
%
% Control Studio A/B,
% The University of Technology Sydney (UTS)
% Sydney, NSW, Australia
%
% Dr Ricardo P. Aguilera
% August 2021
%%%%%%%%%%%%%%%%%%%%%%%%%%%%%%%%%%%%%%%%%%%%%%%%%%%%%%%%%%%%%%%%%%%%%%%%%%%%
function data_out = fcn(data)
    data_out = uC_Tx(data);
end

== matlab function Simulink_Simulink_PIL_Cruise_Crontrol_r2020b/ROCKET/Point Mass with Air Resistance Dynamics /Cd Estimator/Rocket Specific Cd Estimator ==
  data: SA input; Cd output; V input; rho input
function Cd = fcn(SA,V,rho)
u1 =  43.32270126;  % Total rocket SA.
u2 = -0.000687709; % Velocity
u3 = 0.531869262; % Air density
intercept = -0.447146101;
Cd = (SA*u1)+ (V*u2)+ (rho*u3) + (intercept) ;
end

== matlab function Simulink_Simulink_PIL_Cruise_Crontrol_r2020b/Rocket/Point Mass with Air Resistance Dynamics /Cd Estimator/Rocket Specific Cd Estimator ==
  data: SA input; Cd output; V input; rho input
function Cd = fcn(SA,V,rho)
u1 =  43.32270126;  % Total rocket SA.
u2 = -0.000687709; % Velocity
u3 = 0.531869262; % Air density
intercept = -0.447146101;
Cd = (SA*u1)+ (V*u2)+ (rho*u3) + (intercept) ;
end
